simulink model "AIRSPEEDSENSOR"  (R2023b)
settings: Solver=VariableStepAuto  StartTime=0.0  StopTime=10.0  RelTol=1e-3
settings Model: Creator=lucaerviati  LastModifiedBy=monis
settings OptimizationCC: ReuseModelBlockBuffer=off

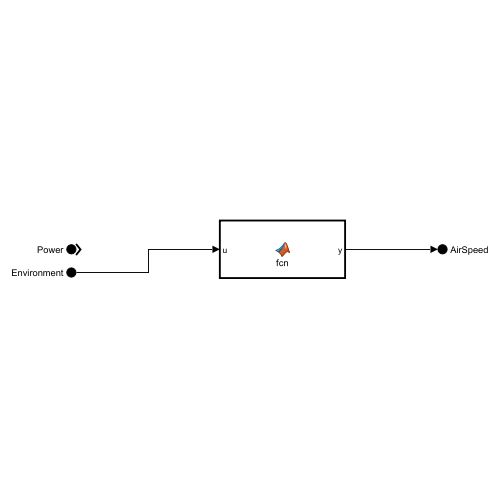
[thumbnail: Simulink's stored preview of the top-level diagram]
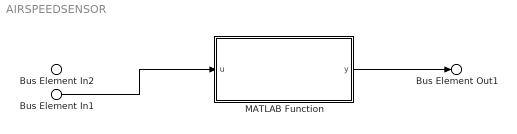
== system AIRSPEEDSENSOR ==
  Bus Element In2 : Inport  PortName=Power
  Bus Element In1 : Inport  Port=2  PortName=Environment
  MATLAB Function : MATLAB Function  TreatAsAtomicUnit=on
  Bus Element Out1 : Outport  PortName=AirSpeed
  wires:
  MATLAB Function/1(y) -> Bus Element Out1/1
  Bus Element In1/1 -> MATLAB Function/1(u)

== matlab function AIRSPEEDSENSOR/MATLAB Function ==
  data: u input; y output
function y = fcn(u)
u = [10,
    9,
    14]
y = u;
